simulink model "Dynamics3"  (R2023b)
settings: Solver=VariableStepAuto  StartTime=0.0  StopTime=300  RelTol=1e-3
undefined symbols (not defined in the file): env, F, iniRoll, initPitch, iniYaw, Light, MIL, tiltIni, uavParam, vIni, xGround, yGround, zGround
libraries: mbdriLib x4, slpidlib x4, aerolibasang x2, aerolibwind2 x2, shared6dof x1, sharedtransform x1, simulink x1, uavutilslib x1
(part 1 of 2)
settings Model: Creator=USER  LastModifiedBy=USER

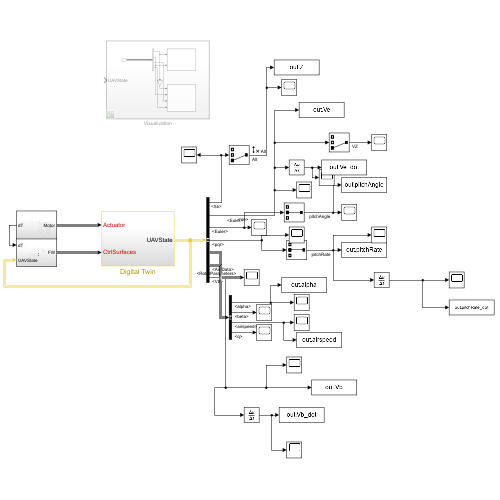
[thumbnail: Simulink's stored preview of the top-level diagram]
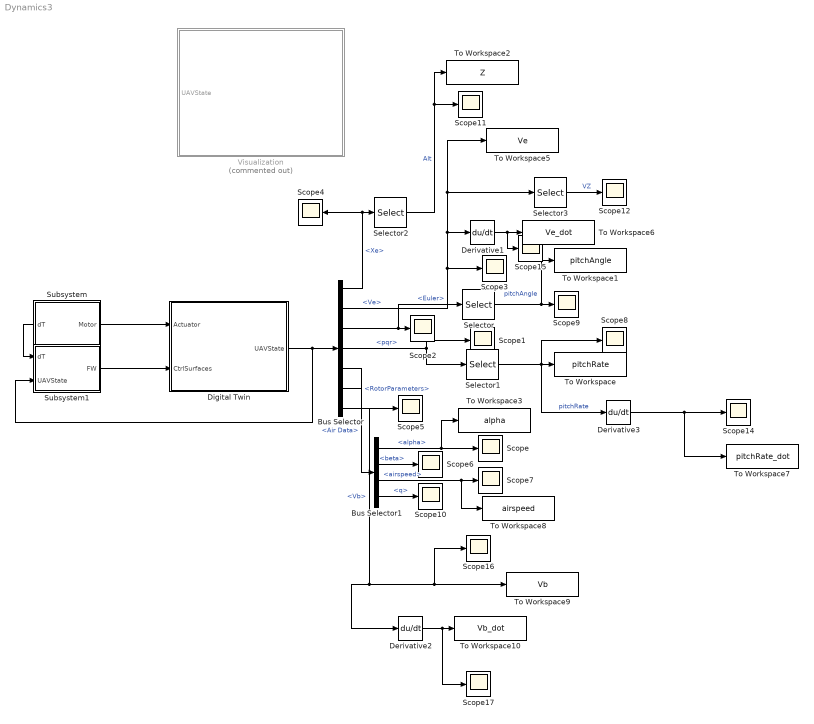
== system Dynamics3 ==
  Bus Selector : BusSelector  OutputSignals=Xe,Ve,Euler,pqr,RotorParameters,Air Data,Vb
  Bus Selector1 : BusSelector  OutputSignals=alpha,beta,airspeed,q
  Derivative1 : Derivative
  Derivative2 : Derivative
  Derivative3 : Derivative
  Digital Twin : Subsystem
  Scope{,1..12,14..17} (17 alike) : Scope
  Selector : Selector  InputPortWidth=3  IndexOptions=Index vector (dialog)  Indices=[2]  OutputSizes=1
  Selector1 : Selector  InputPortWidth=3  IndexOptions=Index vector (dialog)  Indices=[2]  OutputSizes=1
  Selector2 : Selector  InputPortWidth=3  IndexOptions=Index vector (dialog)  Indices=[3]  OutputSizes=1
  Selector3 : Selector  InputPortWidth=3  IndexOptions=Index vector (dialog)  Indices=[3]  OutputSizes=1
  Subsystem : Subsystem
      settings: PortSchema="{\"entries\":[{\"content\":{\"sides\":[{\"content\":{\"connectorIds\":[\"Out2\"]},\"type\":\"ConnectorPlacement.EquallySpacedRectSide\",\"uuid\":\"beef7808-c029-4f06-8f14-a565426224e7\"},{\"content\":{\"connectorIds\":[\"Out1\"],\"side\":\"RIGHT\"},\"type\":\"ConnectorPlacement.EquallySpacedRectSide\",\"uuid\":\"669368ed-0e99-4b02-879e-c65f4105b996\"},{\"content\":{\"side\":\"TOP\"},\"type\":\"ConnectorPlacement.EquallySpacedRectSide\",\"uuid\":\"5dd16cea-975a-4d1b-a565-9c8e907ef411\"}]},\"type\":\"ConnectorPlacement.EquallySpacedConnector\",\"uuid\":\"07c7d036-b657-434c-adc0-0d81d2cf90bb\"}],\"packageUris\":[\"http://schema.mathworks.com/mf0/Connector/R2020b\"],\"version\":\"1.0\"}"
  Subsystem1 : Subsystem
  To Workspace : ToWorkspace  VariableName=pitchRate  SampleTime=-1
  To Workspace1 : ToWorkspace  VariableName=pitchAngle  SampleTime=-1
  To Workspace10 : ToWorkspace  VariableName=Vb_dot  SampleTime=-1
  To Workspace2 : ToWorkspace  VariableName=Z  SampleTime=-1
  To Workspace3 : ToWorkspace  VariableName=alpha  SampleTime=-1
  To Workspace5 : ToWorkspace  VariableName=Ve  SampleTime=-1
  To Workspace6 : ToWorkspace  VariableName=Ve_dot  SampleTime=-1
  To Workspace7 : ToWorkspace  VariableName=pitchRate_dot  SampleTime=-1
  To Workspace8 : ToWorkspace  VariableName=airspeed  SampleTime=-1
  To Workspace9 : ToWorkspace  VariableName=Vb  SampleTime=-1
  Visualization : Subsystem  Commented=on  VariantControl=Visualization==1
  wires:
  Selector1/1 -> To Workspace/1, Scope8/1, Derivative3/1  "pitchRate"
  Bus Selector/3 -> Selector/1, Scope2/1  "<Euler>"
  Selector3/1 -> Scope12/1  "VZ"
  Bus Selector/4 -> Scope1/1, Selector1/1  "<pqr>"
  Digital Twin/1(UAVState) -> Bus Selector/1, Subsystem1/2(UAVState)
  Bus Selector1/4 -> Scope10/1  "<q>"
  Bus Selector1/3 -> To Workspace8/1, Scope7/1  "<airspeed>"
  Derivative1/1 -> Scope15/1, To Workspace6/1
  Subsystem/1(Motor) -> Digital Twin/1(Actuator)
  Bus Selector/7 -> Derivative2/1, Scope16/1, To Workspace9/1  "<Vb>"
  Bus Selector/1 -> Selector2/1, Scope4/1  "<Xe>"
  Bus Selector/5 -> Scope5/1  "<RotorParameters>"
  Bus Selector1/2 -> Scope6/1  "<beta>"
  Selector/1 -> To Workspace1/1, Scope9/1  "pitchAngle"
  Bus Selector1/1 -> To Workspace3/1, Scope/1  "<alpha>"
  Bus Selector/2 -> Derivative1/1, To Workspace5/1, Selector3/1, Scope3/1  "<Ve>"
  Selector2/1 -> To Workspace2/1, Scope11/1  "Alt"
  Derivative2/1 -> Scope17/1, To Workspace10/1
  Subsystem1/1(FW) -> Digital Twin/2(CtrlSurfaces)
  Bus Selector/6 -> Bus Selector1/1  "<Air Data>"
  Derivative3/1 -> Scope14/1, To Workspace7/1
  Subsystem/2(dT) -> Subsystem1/1(dT)

== system Dynamics3/Digital Twin ==
  Actuator : Inport
  CtrlSurfaces : Inport  Port=2
  6DOF (Euler Angles)1 : shared6dof/6DOF (Euler Angles)  units=Metric (MKS)  mtype=Fixed  rep=Euler Angles  xme_0=[xGround, yGround, zGround]  Vm_0=[vIni 0 0]  eul_0=[iniRoll initPitch iniYaw]  pm_0=[0 0 0]  mass_0=6.031  mass_e=0.5  mass_f=2.0  inertia=[uavParam.geom.Ixx 0 0; 0 uavParam.geom.Iyy 0; 0 0 uavParam.geom.Izz]  inertia_e=eye(3)  inertia_f=2*eye(3)  k_quat=1.0  vre_flag=on  abi_flag=on  aMode=0  xme_statename=''  Vm_statename=''  eul_statename=''  quat_statename=''  pm_statename=''  mass_statename=''
  Bus Selector : BusSelector  OutputSignals=RotorParameters.w1,RotorParameters.w2,RotorParameters.w3,RotorParameters.w4
  Force and Moments : Subsystem
  Ground Truth Bus : Subsystem
  Scope : Scope  NumInputPorts=4
  Terminator : Terminator
  UAVState : Outport
  wires:
  Bus Selector/4 -> Scope/4  "<w4>"
  Bus Selector/3 -> Scope/3  "<w3>"
  Bus Selector/2 -> Scope/2  "<w2>"
  Bus Selector/1 -> Scope/1  "<w1>"
  Ground Truth Bus/1(Ground Truth) -> Force and Moments/3(States), UAVState/1, Bus Selector/1  "Ground Truth"
  6DOF (Euler Angles)1/9 -> Ground Truth Bus/8(Abe)
  Force and Moments/4(AirData) -> Ground Truth Bus/10(AirData)
  Force and Moments/3(RotorParams) -> Ground Truth Bus/9(RotorParams)  "RotorParams"
  6DOF (Euler Angles)1/8 -> Ground Truth Bus/7(Abb)  "Abb"
  6DOF (Euler Angles)1/6 -> Ground Truth Bus/6(pqr)  "pqr"
  6DOF (Euler Angles)1/5 -> Ground Truth Bus/5(Vb)  "Vb"
  6DOF (Euler Angles)1/4 -> Ground Truth Bus/4(DCMbe)  "DCMbe"
  6DOF (Euler Angles)1/3 -> Ground Truth Bus/3(Euler)  "Euler"
  6DOF (Euler Angles)1/2 -> Ground Truth Bus/2(Xe)  "Xe"
  6DOF (Euler Angles)1/1 -> Ground Truth Bus/1(Ve)  "Ve"
  CtrlSurfaces/1 -> Force and Moments/2(CtrlSurfaces)
  Actuator/1 -> Force and Moments/1(Actuator)
  Force and Moments/2(M) -> 6DOF (Euler Angles)1/2
  Force and Moments/1(F) -> 6DOF (Euler Angles)1/1
  6DOF (Euler Angles)1/7 -> Terminator/1

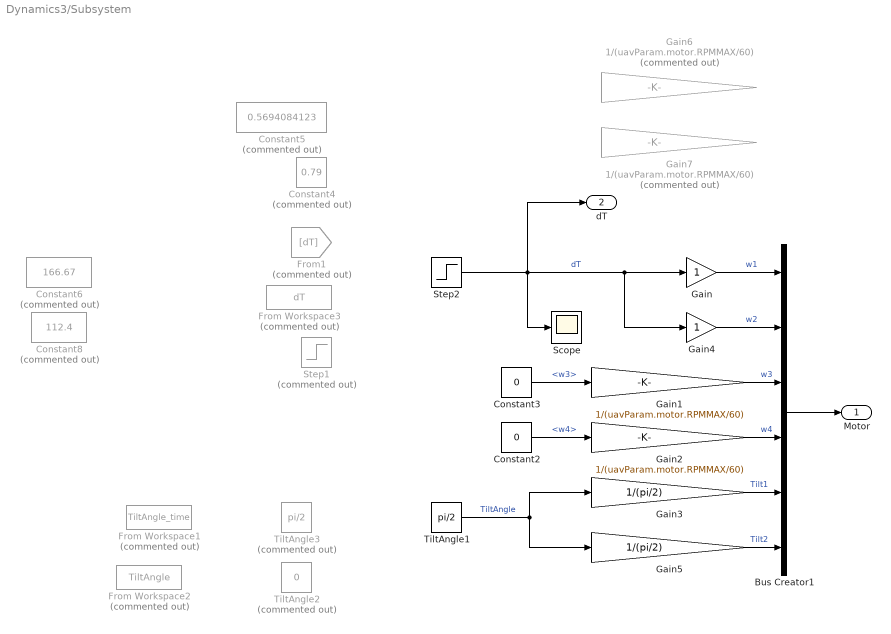
== system Dynamics3/Subsystem ==
  Bus Creator1 : BusCreator  Inputs=6  OutDataTypeStr=Bus: RotorCntrlBus
  Constant2 : Constant  Value=0
  Constant3 : Constant  Value=0
  Constant4 : Constant  Commented=on  Value=0.79
  Constant5 : Constant  Commented=on  Value=0.5694084123
  Constant6 : Constant  Commented=on  Value=166.67
  Constant8 : Constant  Commented=on  Value=112.4
  From Workspace1 : FromWorkspace  Commented=on  VariableName=TiltAngle_time
  From Workspace2 : FromWorkspace  Commented=on  VariableName=TiltAngle
  From Workspace3 : FromWorkspace  Commented=on  VariableName=dT
  From1 : From  Commented=on  GotoTag=dT
  Gain : Gain
  Gain1 : Gain  Gain=1/(uavParam.motor.RPMMAX/60)
  Gain2 : Gain  Gain=1/(uavParam.motor.RPMMAX/60)
  Gain3 : Gain  Gain=1/(pi/2)
  Gain4 : Gain
  Gain5 : Gain  Gain=1/(pi/2)
  Gain6 : Gain  Commented=on  Gain=1/(uavParam.motor.RPMMAX/60)
  Gain7 : Gain  Commented=on  Gain=1/(uavParam.motor.RPMMAX/60)
  Scope : Scope
  Step1 : Step  Commented=on  Time=100  Before=0.79  After=0.5694084123  SampleTime=0
  Step2 : Step  Time=100  Before=0.79  After=0.5694084123  SampleTime=0
  TiltAngle1 : Constant  Value=pi/2
  TiltAngle2 : Constant  Commented=on  Value=0
  TiltAngle3 : Constant  Commented=on  Value=pi/2
  Motor : Outport
  dT : Outport  Port=2
  wires:
  Constant3/1 -> Gain1/1  "<w3>"
  Constant2/1 -> Gain2/1  "<w4>"
  Gain5/1 -> Bus Creator1/6  "Tilt2"
  Gain3/1 -> Bus Creator1/5  "Tilt1"
  Gain1/1 -> Bus Creator1/3  "w3"
  Gain2/1 -> Bus Creator1/4  "w4"
  TiltAngle1/1 -> Gain5/1, Gain3/1  "TiltAngle"
  Bus Creator1/1 -> Motor/1
  Gain4/1 -> Bus Creator1/2  "w2"
  Gain/1 -> Bus Creator1/1  "w1"
  Step2/1 -> dT/1, Scope/1, Gain4/1, Gain/1  "dT"

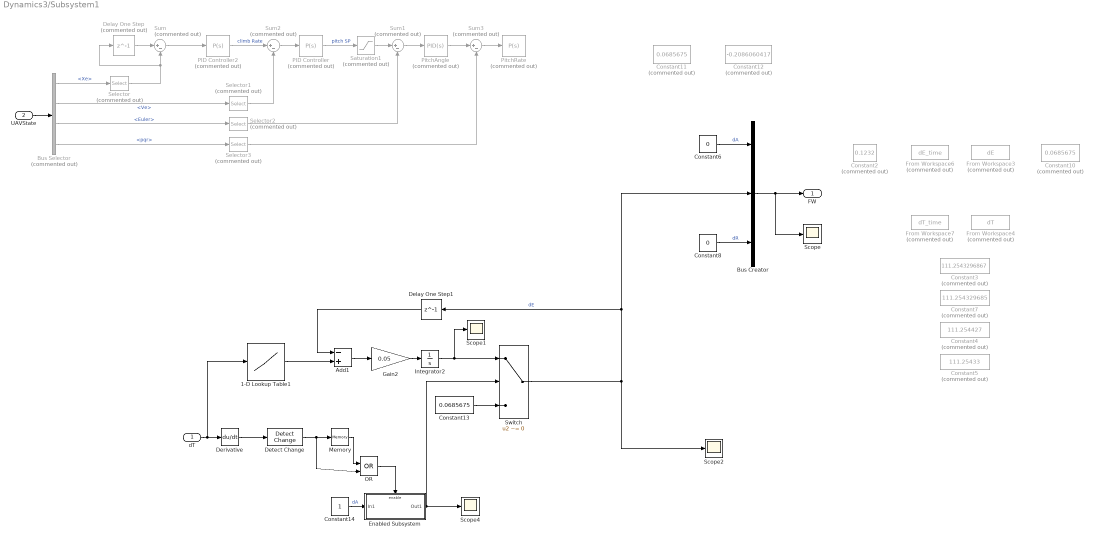
== system Dynamics3/Subsystem1 ==
  dT : Inport
  UAVState : Inport  Port=2
  1-D Lookup Table1 : Lookup_n-D  NumberOfTableDimensions=1  BreakpointsForDimension1=[0.5694084123;0.79]  Table=[-0.2086060417;0.0685675]  InternalRulePriority=Speed  RndMeth=Simplest
  Add1 : Sum  Inputs=-+
  Bus Creator : BusCreator  Inputs=3
  Bus Selector : BusSelector  Commented=on  OutputSignals=Xe,Ve,Euler,pqr
  Constant10 : Constant  Commented=on  Value=0.0685675
  Constant11 : Constant  Commented=on  Value=0.0685675
  Constant12 : Constant  Commented=on  Value=-0.2086060417
  Constant13 : Constant  Value=0.0685675
  Constant14 : Constant
  Constant2 : Constant  Commented=on  Value=0.1232
  Constant3 : Constant  Commented=on  Value=111.2543296867
  Constant4 : Constant  Commented=on  Value=111.254427
  Constant5 : Constant  Commented=on  Value=111.25433
  Constant6 : Constant  Value=0
  Constant7 : Constant  Commented=on  Value=111.254329685
  Constant8 : Constant  Value=0
  Delay One Step : Delay  Commented=on  DelayLength=1
  Delay One Step1 : Delay  DelayLength=1
  Derivative : Derivative
  Detect Change : simulink/Logic and Bit Operations/Detect Change  vinit=0  OutDataTypeStr=boolean
  Enabled Subsystem : Subsystem  TreatAsAtomicUnit=on
  From Workspace3 : FromWorkspace  Commented=on  VariableName=dE  OutDataTypeStr=double
  From Workspace4 : FromWorkspace  Commented=on  VariableName=dT  OutDataTypeStr=double
  From Workspace6 : FromWorkspace  Commented=on  VariableName=dE_time
  From Workspace7 : FromWorkspace  Commented=on  VariableName=dT_time
  Gain2 : Gain  Gain=0.05
  Integrator2 : Integrator
  Memory : Memory
  OR : Logic  Operator=OR  IconShape=distinctive  AllPortsSameDT=off  OutDataTypeStr=boolean
  PID Controller : slpidlib/PID Controller  Commented=on  Controller=P  Form=Parallel  TimeDomain=Continuous-time  UseExternalTs=off  SampleTime=-1  IntegratorMethod=Forward Euler  FilterMethod=Forward Euler  ControllerParametersSource=internal  P=0.253636873440471  I=1  UseKiTs=off  D=0  N=100  UseFilter=on  TunerSelectOption=Transfer Function Based (PID Tuner App)  InitialConditionSource=internal  InitialConditionForIntegrator=0  InitialConditionForFilter=0  DifferentiatorICPrevScaledInput=0  ExternalReset=none  TrackingMode=off  Kt=1  LimitOutput=off  SatLimitsSource=internal  UpperSaturationLimit=inf  LowerSaturationLimit=-inf  LinearizeAsGain=on  AntiWindupMode=none  Kb=1  LimitIntegrator=off  UpperIntegratorSaturationLimit=inf  LowerIntegratorSaturationLimit=-inf  POutMin=[]  POutMax=[]  IOutMin=[]  IOutMax=[]  DOutMin=[]  DOutMax=[]  NOutMin=[]  NOutMax=[]  SumOutMin=[]  SumOutMax=[]  SaturationOutMin=[]  SaturationOutMax=[]  PParamMin=[]  PParamMax=[]  IParamMin=[]  IParamMax=[]  DParamMin=[]  DParamMax=[]  NParamMin=[]  NParamMax=[]  KbParamMin=[]  KbParamMax=[]  KtParamMin=[]  KtParamMax=[]  KbOutMin=[]  KbOutMax=[]  KtOutMin=[]  KtOutMax=[]  IntegratorOutMin=[]  IntegratorOutMax=[]  FilterOutMin=[]  FilterOutMax=[]  SumI1OutMin=[]  SumI1OutMax=[]  SumI2OutMin=[]  SumI2OutMax=[]  SumI3OutMin=[]  SumI3OutMax=[]  SumI4OutMin=[]  SumI4OutMax=[]  SumDOutMin=[]  SumDOutMax=[]  DifferentiatorOutMin=[]  DifferentiatorOutMax=[]  FilterDiffOutCoefMin=[]  FilterDiffOutCoefMax=[]  ReciprocalOutMin=[]  ReciprocalOutMax=[]  SumDenOutMin=[]  SumDenOutMax=[]  SumNumOutMin=[]  SumNumOutMax=[]  DivideOutMin=[]  DivideOutMax=[]  UdiffTsProdOutMin=[]  UdiffTsProdOutMax=[]  NTsProdOutMin=[]  NTsProdOutMax=[]  UintegralTsProdOutMin=[]  UintegralTsProdOutMax=[]  UngainTsProdOutMin=[]  UngainTsProdOutMax=[]  ClampingZeroOutDataTypeStr=Inherit: Inherit via back propagation  ClampingZeroOutMin=[]  ClampingZeroOutMax=[]  FilterDenConstantOutDataTypeStr=Inherit: Inherit via back propagation  FilterDenConstantOutMin=[]  FilterDenConstantOutMax=[]  PCopyOutDataTypeStr=Inherit: Inherit via back propagation  PCopyOutMin=[]  PCopyOutMax=[]  NCopyOutDataTypeStr=Inherit: Inherit via back propagation  NCopyOutMin=[]  NCopyOutMax=[]  IntegratorContinuousStateAttributes=''  IntegratorStateMustResolveToSignalObject=off  IntegratorRTWStateStorageClass=Auto  FilterContinuousStateAttributes=''  FilterStateMustResolveToSignalObject=off  FilterRTWStateStorageClass=Auto  ParallelPVariant=InternalParameters  IdealPVariant=Disabled  IVariant=Disabled  DVariant=Disabled  IntegratorVariant=Disabled  SatVariant=Disabled  AWVariant=Disabled  PCopyVariant=Disabled  TRVariant=Disabled  FdbkBlocksVariant=Forward  IdealPFdbkVariant=Disabled  SatFdbkVariant=Disabled  DerivativeFilterVariant=Disabled  NVariant=Disabled  NCopyVariant=Disabled_SignalSpec  FilterICVariant=Disabled  IntegratorICVariant=Disabled  ExternalResetVariant=Disabled  TRSumVariant=Passthrough  SumFdbkVariant=Disabled  SumVariant=Passthrough_P  TsampFilterVariant=InternalTs  TsampNgainVariant=Passthrough  TsampIntegralVariant=Disabled_SignalSpec  ExternalSaturationOutDataTypeStr=Inherit: Same as second input
  PID Controller2 : slpidlib/PID Controller  Commented=on  Controller=P  Form=Parallel  TimeDomain=Continuous-time  UseExternalTs=off  SampleTime=-1  IntegratorMethod=Forward Euler  FilterMethod=Forward Euler  ControllerParametersSource=internal  P=100  I=1  UseKiTs=off  D=0  N=100  UseFilter=on  TunerSelectOption=Transfer Function Based (PID Tuner App)  InitialConditionSource=internal  InitialConditionForIntegrator=0  InitialConditionForFilter=0  DifferentiatorICPrevScaledInput=0  ExternalReset=none  TrackingMode=off  Kt=1  LimitOutput=off  SatLimitsSource=internal  UpperSaturationLimit=inf  LowerSaturationLimit=-inf  LinearizeAsGain=on  AntiWindupMode=none  Kb=1  LimitIntegrator=off  UpperIntegratorSaturationLimit=inf  LowerIntegratorSaturationLimit=-inf  POutMin=[]  POutMax=[]  IOutMin=[]  IOutMax=[]  DOutMin=[]  DOutMax=[]  NOutMin=[]  NOutMax=[]  SumOutMin=[]  SumOutMax=[]  SaturationOutMin=[]  SaturationOutMax=[]  PParamMin=[]  PParamMax=[]  IParamMin=[]  IParamMax=[]  DParamMin=[]  DParamMax=[]  NParamMin=[]  NParamMax=[]  KbParamMin=[]  KbParamMax=[]  KtParamMin=[]  KtParamMax=[]  KbOutMin=[]  KbOutMax=[]  KtOutMin=[]  KtOutMax=[]  IntegratorOutMin=[]  IntegratorOutMax=[]  FilterOutMin=[]  FilterOutMax=[]  SumI1OutMin=[]  SumI1OutMax=[]  SumI2OutMin=[]  SumI2OutMax=[]  SumI3OutMin=[]  SumI3OutMax=[]  SumI4OutMin=[]  SumI4OutMax=[]  SumDOutMin=[]  SumDOutMax=[]  DifferentiatorOutMin=[]  DifferentiatorOutMax=[]  FilterDiffOutCoefMin=[]  FilterDiffOutCoefMax=[]  ReciprocalOutMin=[]  ReciprocalOutMax=[]  SumDenOutMin=[]  SumDenOutMax=[]  SumNumOutMin=[]  SumNumOutMax=[]  DivideOutMin=[]  DivideOutMax=[]  UdiffTsProdOutMin=[]  UdiffTsProdOutMax=[]  NTsProdOutMin=[]  NTsProdOutMax=[]  UintegralTsProdOutMin=[]  UintegralTsProdOutMax=[]  UngainTsProdOutMin=[]  UngainTsProdOutMax=[]  ClampingZeroOutDataTypeStr=Inherit: Inherit via back propagation  ClampingZeroOutMin=[]  ClampingZeroOutMax=[]  FilterDenConstantOutDataTypeStr=Inherit: Inherit via back propagation  FilterDenConstantOutMin=[]  FilterDenConstantOutMax=[]  PCopyOutDataTypeStr=Inherit: Inherit via back propagation  PCopyOutMin=[]  PCopyOutMax=[]  NCopyOutDataTypeStr=Inherit: Inherit via back propagation  NCopyOutMin=[]  NCopyOutMax=[]  IntegratorContinuousStateAttributes=''  IntegratorStateMustResolveToSignalObject=off  IntegratorRTWStateStorageClass=Auto  FilterContinuousStateAttributes=''  FilterStateMustResolveToSignalObject=off  FilterRTWStateStorageClass=Auto  ParallelPVariant=InternalParameters  IdealPVariant=Disabled  IVariant=Disabled  DVariant=Disabled  IntegratorVariant=Disabled  SatVariant=Disabled  AWVariant=Disabled  PCopyVariant=Disabled  TRVariant=Disabled  FdbkBlocksVariant=Forward  IdealPFdbkVariant=Disabled  SatFdbkVariant=Disabled  DerivativeFilterVariant=Disabled  NVariant=Disabled  NCopyVariant=Disabled_SignalSpec  FilterICVariant=Disabled  IntegratorICVariant=Disabled  ExternalResetVariant=Disabled  TRSumVariant=Passthrough  SumFdbkVariant=Disabled  SumVariant=Passthrough_P  TsampFilterVariant=InternalTs  TsampNgainVariant=Passthrough  TsampIntegralVariant=Disabled_SignalSpec  ExternalSaturationOutDataTypeStr=Inherit: Same as second input
  PitchAngle : slpidlib/PID Controller  Commented=on  Controller=PID  Form=Parallel  TimeDomain=Continuous-time  UseExternalTs=off  SampleTime=-1  IntegratorMethod=Forward Euler  FilterMethod=Forward Euler  ControllerParametersSource=internal  P=17.6399272009125  I=10.1914925604101  UseKiTs=off  D=1.4272793655692  N=0.16530941788163  UseFilter=on  TunerSelectOption=Transfer Function Based (PID Tuner App)  InitialConditionSource=internal  InitialConditionForIntegrator=0  InitialConditionForFilter=0  DifferentiatorICPrevScaledInput=0  ExternalReset=none  TrackingMode=off  Kt=1  LimitOutput=off  SatLimitsSource=internal  UpperSaturationLimit=inf  LowerSaturationLimit=-inf  LinearizeAsGain=on  AntiWindupMode=none  Kb=1  LimitIntegrator=off  UpperIntegratorSaturationLimit=inf  LowerIntegratorSaturationLimit=-inf  POutMin=[]  POutMax=[]  IOutMin=[]  IOutMax=[]  DOutMin=[]  DOutMax=[]  NOutMin=[]  NOutMax=[]  SumOutMin=[]  SumOutMax=[]  SaturationOutMin=[]  SaturationOutMax=[]  PParamMin=[]  PParamMax=[]  IParamMin=[]  IParamMax=[]  DParamMin=[]  DParamMax=[]  NParamMin=[]  NParamMax=[]  KbParamMin=[]  KbParamMax=[]  KtParamMin=[]  KtParamMax=[]  KbOutMin=[]  KbOutMax=[]  KtOutMin=[]  KtOutMax=[]  IntegratorOutMin=[]  IntegratorOutMax=[]  FilterOutMin=[]  FilterOutMax=[]  SumI1OutMin=[]  SumI1OutMax=[]  SumI2OutMin=[]  SumI2OutMax=[]  SumI3OutMin=[]  SumI3OutMax=[]  SumI4OutMin=[]  SumI4OutMax=[]  SumDOutMin=[]  SumDOutMax=[]  DifferentiatorOutMin=[]  DifferentiatorOutMax=[]  FilterDiffOutCoefMin=[]  FilterDiffOutCoefMax=[]  ReciprocalOutMin=[]  ReciprocalOutMax=[]  SumDenOutMin=[]  SumDenOutMax=[]  SumNumOutMin=[]  SumNumOutMax=[]  DivideOutMin=[]  DivideOutMax=[]  UdiffTsProdOutMin=[]  UdiffTsProdOutMax=[]  NTsProdOutMin=[]  NTsProdOutMax=[]  UintegralTsProdOutMin=[]  UintegralTsProdOutMax=[]  UngainTsProdOutMin=[]  UngainTsProdOutMax=[]  ClampingZeroOutDataTypeStr=Inherit: Inherit via back propagation  ClampingZeroOutMin=[]  ClampingZeroOutMax=[]  FilterDenConstantOutDataTypeStr=Inherit: Inherit via back propagation  FilterDenConstantOutMin=[]  FilterDenConstantOutMax=[]  PCopyOutDataTypeStr=Inherit: Inherit via back propagation  PCopyOutMin=[]  PCopyOutMax=[]  NCopyOutDataTypeStr=Inherit: Inherit via back propagation  NCopyOutMin=[]  NCopyOutMax=[]  IntegratorContinuousStateAttributes=''  IntegratorStateMustResolveToSignalObject=off  IntegratorRTWStateStorageClass=Auto  FilterContinuousStateAttributes=''  FilterStateMustResolveToSignalObject=off  FilterRTWStateStorageClass=Auto  ParallelPVariant=InternalParameters  IdealPVariant=Disabled  IVariant=InternalParameters  DVariant=InternalParameters  IntegratorVariant=Continuous  SatVariant=Disabled  AWVariant=Passthrough  PCopyVariant=Disabled  TRVariant=Disabled  FdbkBlocksVariant=Forward  IdealPFdbkVariant=Disabled  SatFdbkVariant=Disabled  DerivativeFilterVariant=ContFilter  NVariant=InternalParameters  NCopyVariant=Disabled  FilterICVariant=InternalICsFilter  IntegratorICVariant=InternalICs  ExternalResetVariant=Disabled  TRSumVariant=Passthrough  SumFdbkVariant=Disabled  SumVariant=Sum_PID  TsampFilterVariant=InternalTs  TsampNgainVariant=Passthrough  TsampIntegralVariant=Disabled_SignalSpec  ExternalSaturationOutDataTypeStr=Inherit: Same as second input
  PitchRate : slpidlib/PID Controller  Commented=on  Controller=P  Form=Parallel  TimeDomain=Continuous-time  UseExternalTs=off  SampleTime=-1  IntegratorMethod=Forward Euler  FilterMethod=Forward Euler  ControllerParametersSource=internal  P=0.198532533167891  I=1  UseKiTs=off  D=0  N=100  UseFilter=on  TunerSelectOption=Transfer Function Based (PID Tuner App)  InitialConditionSource=internal  InitialConditionForIntegrator=0  InitialConditionForFilter=0  DifferentiatorICPrevScaledInput=0  ExternalReset=none  TrackingMode=off  Kt=1  LimitOutput=off  SatLimitsSource=internal  UpperSaturationLimit=inf  LowerSaturationLimit=-inf  LinearizeAsGain=on  AntiWindupMode=none  Kb=1  LimitIntegrator=off  UpperIntegratorSaturationLimit=inf  LowerIntegratorSaturationLimit=-inf  POutMin=[]  POutMax=[]  IOutMin=[]  IOutMax=[]  DOutMin=[]  DOutMax=[]  NOutMin=[]  NOutMax=[]  SumOutMin=[]  SumOutMax=[]  SaturationOutMin=[]  SaturationOutMax=[]  PParamMin=[]  PParamMax=[]  IParamMin=[]  IParamMax=[]  DParamMin=[]  DParamMax=[]  NParamMin=[]  NParamMax=[]  KbParamMin=[]  KbParamMax=[]  KtParamMin=[]  KtParamMax=[]  KbOutMin=[]  KbOutMax=[]  KtOutMin=[]  KtOutMax=[]  IntegratorOutMin=[]  IntegratorOutMax=[]  FilterOutMin=[]  FilterOutMax=[]  SumI1OutMin=[]  SumI1OutMax=[]  SumI2OutMin=[]  SumI2OutMax=[]  SumI3OutMin=[]  SumI3OutMax=[]  SumI4OutMin=[]  SumI4OutMax=[]  SumDOutMin=[]  SumDOutMax=[]  DifferentiatorOutMin=[]  DifferentiatorOutMax=[]  FilterDiffOutCoefMin=[]  FilterDiffOutCoefMax=[]  ReciprocalOutMin=[]  ReciprocalOutMax=[]  SumDenOutMin=[]  SumDenOutMax=[]  SumNumOutMin=[]  SumNumOutMax=[]  DivideOutMin=[]  DivideOutMax=[]  UdiffTsProdOutMin=[]  UdiffTsProdOutMax=[]  NTsProdOutMin=[]  NTsProdOutMax=[]  UintegralTsProdOutMin=[]  UintegralTsProdOutMax=[]  UngainTsProdOutMin=[]  UngainTsProdOutMax=[]  ClampingZeroOutDataTypeStr=Inherit: Inherit via back propagation  ClampingZeroOutMin=[]  ClampingZeroOutMax=[]  FilterDenConstantOutDataTypeStr=Inherit: Inherit via back propagation  FilterDenConstantOutMin=[]  FilterDenConstantOutMax=[]  PCopyOutDataTypeStr=Inherit: Inherit via back propagation  PCopyOutMin=[]  PCopyOutMax=[]  NCopyOutDataTypeStr=Inherit: Inherit via back propagation  NCopyOutMin=[]  NCopyOutMax=[]  IntegratorContinuousStateAttributes=''  IntegratorStateMustResolveToSignalObject=off  IntegratorRTWStateStorageClass=Auto  FilterContinuousStateAttributes=''  FilterStateMustResolveToSignalObject=off  FilterRTWStateStorageClass=Auto  ParallelPVariant=InternalParameters  IdealPVariant=Disabled  IVariant=Disabled  DVariant=Disabled  IntegratorVariant=Disabled  SatVariant=Disabled  AWVariant=Disabled  PCopyVariant=Disabled  TRVariant=Disabled  FdbkBlocksVariant=Forward  IdealPFdbkVariant=Disabled  SatFdbkVariant=Disabled  DerivativeFilterVariant=Disabled  NVariant=Disabled  NCopyVariant=Disabled_SignalSpec  FilterICVariant=Disabled  IntegratorICVariant=Disabled  ExternalResetVariant=Disabled  TRSumVariant=Passthrough  SumFdbkVariant=Disabled  SumVariant=Passthrough_P  TsampFilterVariant=InternalTs  TsampNgainVariant=Passthrough  TsampIntegralVariant=Disabled_SignalSpec  ExternalSaturationOutDataTypeStr=Inherit: Same as second input
  Saturation1 : Saturate  Commented=on  UpperLimit=0.17  LowerLimit=-0.17
  Scope{,1..2,4} (4 alike) : Scope
  Selector : Selector  Commented=on  InputPortWidth=3  IndexOptions=Index vector (dialog)  Indices=3  OutputSizes=1
  Selector1 : Selector  Commented=on  InputPortWidth=3  IndexOptions=Index vector (dialog)  Indices=3  OutputSizes=1
  Selector2 : Selector  Commented=on  InputPortWidth=3  IndexOptions=Index vector (dialog)  Indices=2  OutputSizes=1
  Selector3 : Selector  Commented=on  InputPortWidth=3  IndexOptions=Index vector (dialog)  Indices=2  OutputSizes=1
  Sum{,1..3} (4 alike) : Sum  Commented=on  Inputs=|+-
  Switch : Switch  Criteria=u2 ~= 0  SaturateOnIntegerOverflow=off  InputSameDT=off
  FW : Outport
  wires:
  Constant6/1 -> Bus Creator/1  "dA"
  Constant8/1 -> Bus Creator/3  "dR"
  Bus Creator/1 -> Scope/1, FW/1
  Delay One Step/1 -> Sum/1
  Selector/1 -> Delay One Step/1, Sum/2
  Sum/1 -> PID Controller2/1
  Bus Selector/1 -> Selector/1  "<Xe>"
  PID Controller/1 -> Saturation1/1  "pitch SP"
  Bus Selector/2 -> Selector1/1  "<Ve>"
  Selector1/1 -> Sum2/2
  PID Controller2/1 -> Sum2/1  "climb Rate"
  Sum2/1 -> PID Controller/1
  Bus Selector/3 -> Selector2/1  "<Euler>"
  Bus Selector/4 -> Selector3/1  "<pqr>"
  Saturation1/1 -> Sum1/1
  Sum1/1 -> PitchAngle/1
  PitchAngle/1 -> Sum3/1
  Sum3/1 -> PitchRate/1
  Selector2/1 -> Sum1/2
  Selector3/1 -> Sum3/2
  Switch/1 -> Delay One Step1/1, Bus Creator/2, Scope2/1  "dE"
  Enabled Subsystem/1(Out1) -> Switch/2, Scope4/1
  Derivative/1 -> Detect Change/1
  Detect Change/1 -> Memory/1, OR/2
  Memory/1 -> OR/1
  OR/1 -> Enabled Subsystem/Enable
  Constant13/1 -> Switch/3
  Constant14/1 -> Enabled Subsystem/1(In1)  "dA"
  UAVState/1 -> Bus Selector/1
  Gain2/1 -> Integrator2/1
  Integrator2/1 -> Scope1/1, Switch/1
  Add1/1 -> Gain2/1
  1-D Lookup Table1/1 -> Add1/2
  dT/1 -> 1-D Lookup Table1/1, Derivative/1
  Delay One Step1/1 -> Add1/1

== system Dynamics3/Visualization ==
  UAVState : Inport
  Bus Selector : BusSelector  OutputSignals=Xe,q,RotorParameters.Rotor A,RotorParameters.Rotor B
  Gain : Gain  Gain=0
  Subsystem : Subsystem
  Trajectory : uavutilslib/UAV Animation  UAVType=FixedWing  UAVSize=5  InertialZDirection=Down  SampleTime=0.1
  wires:
  Bus Selector/4 -> Subsystem/4(RotorB)  "<Rotor B>"
  Bus Selector/3 -> Subsystem/3(RotorA)  "<Rotor A>"
  UAVState/1 -> Bus Selector/1
  Gain/1 -> Subsystem/1(<Xe>)
  Bus Selector/1 -> Gain/1, Trajectory/1  "<Xe>"
  Bus Selector/2 -> Trajectory/2, Subsystem/2(<q>)  "<q>"

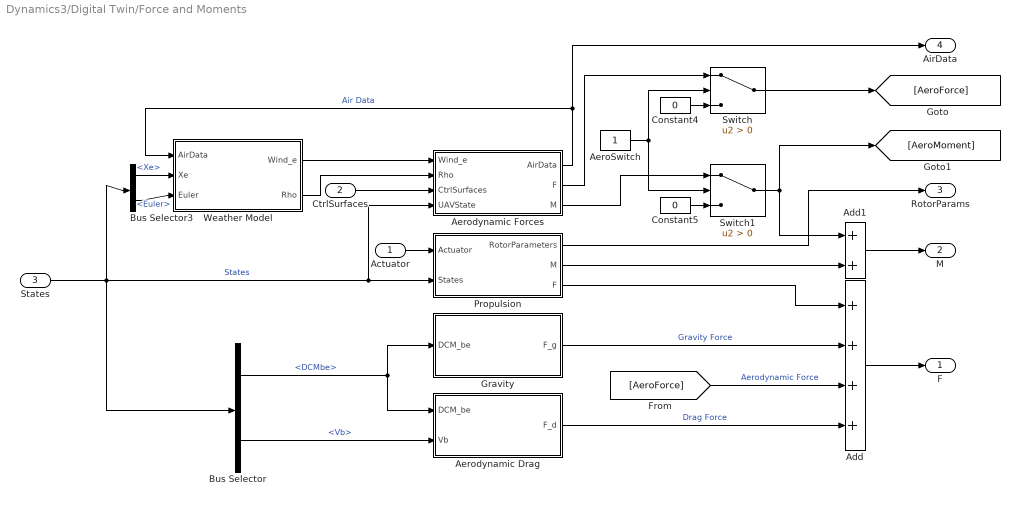
== system Dynamics3/Digital Twin/Force and Moments ==
  Actuator : Inport
  CtrlSurfaces : Inport  Port=2
  States : Inport  Port=3
  Add : Sum  Inputs=++++
  Add1 : Sum
  AeroSwitch : Constant
  Aerodynamic Drag : Subsystem
  Aerodynamic Forces : Subsystem
  Bus Selector : BusSelector  OutputSignals=DCMbe,Vb
  Bus Selector3 : BusSelector  OutputSignals=Xe,Euler
  Constant4 : Constant  Value=0
  Constant5 : Constant  Value=0
  Gravity : Subsystem
  Propulsion : Subsystem
  Switch : Switch  Criteria=u2 > Threshold  SaturateOnIntegerOverflow=off  InputSameDT=off
  Switch1 : Switch  Criteria=u2 > Threshold  SaturateOnIntegerOverflow=off  InputSameDT=off
  Weather Model : Subsystem  Variant=on  VariantControl=Weather Model
  F : Outport
  M : Outport  Port=2
  RotorParams : Outport  Port=3
  AirData : Outport  Port=4
  wires:
  Weather Model/2(Rho) -> Aerodynamic Forces/2(Rho)
  Weather Model/1(Wind_e) -> Aerodynamic Forces/1(Wind_e)
  Bus Selector3/2 -> Weather Model/3(Euler)  "<Euler>"
  Bus Selector3/1 -> Weather Model/2(Xe)  "<Xe>"
  Aerodynamic Forces/1(AirData) -> Weather Model/1(AirData), AirData/1  "Air Data"
  Propulsion/1(RotorParameters) -> RotorParams/1
  Actuator/1 -> Propulsion/1(Actuator)
  Aerodynamic Forces/3(M) -> Switch1/1
  Switch1/1 -> [AeroMoment], Add1/1
  Constant5/1 -> Switch1/3
  AeroSwitch/1 -> Switch1/2, Switch/2
  Constant4/1 -> Switch/3
  Switch/1 -> [AeroForce]
  Aerodynamic Forces/2(F) -> Switch/1
  [AeroForce] -> Add/3  "Aerodynamic Force"
  Propulsion/2(M) -> Add1/2
  Add1/1 -> M/1
  CtrlSurfaces/1 -> Aerodynamic Forces/3(CtrlSurfaces)
  States/1 -> Propulsion/2(States), Aerodynamic Forces/4(UAVState), Bus Selector/1, Bus Selector3/1  "States"
  Add/1 -> F/1
  Bus Selector/2 -> Aerodynamic Drag/2(Vb)  "<Vb>"
  Aerodynamic Drag/1(F_d) -> Add/4  "Drag Force"
  Gravity/1(F_g) -> Add/2  "Gravity Force"
  Propulsion/3(F) -> Add/1
  Bus Selector/1 -> Aerodynamic Drag/1(DCM_be), Gravity/1(DCM_be)  "<DCMbe>"

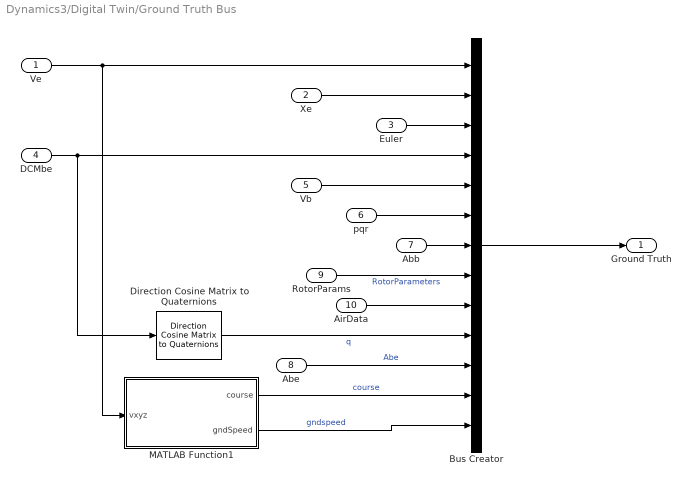
== system Dynamics3/Digital Twin/Ground Truth Bus ==
  Ve : Inport
  Xe : Inport  Port=2
  Euler : Inport  Port=3
  DCMbe : Inport  Port=4
  Vb : Inport  Port=5
  pqr : Inport  Port=6
  Abb : Inport  Port=7
  Abe : Inport  Port=8
  RotorParams : Inport  Port=9
  AirData : Inport  Port=10
  Bus Creator : BusCreator  Inputs=13
  Direction Cosine Matrix to Quaternions : sharedtransform/Direction Cosine Matrix  to Quaternions  aMode=0  action=None  tolerance=eps(2)
      settings: LibrarySourceBlock=|
      | aerolibtransform2/Direction Cosine Matrix
      | to Quaternions
  MATLAB Function1 : MATLAB Function  TreatAsAtomicUnit=on
  Ground Truth : Outport
  wires:
  Ve/1 -> Bus Creator/1, MATLAB Function1/1(vxyz)
  MATLAB Function1/1(course) -> Bus Creator/12  "course"
  MATLAB Function1/2(gndSpeed) -> Bus Creator/13  "gndspeed"
  Abe/1 -> Bus Creator/11  "Abe"
  RotorParams/1 -> Bus Creator/8  "RotorParameters"
  Direction Cosine Matrix to Quaternions/1 -> Bus Creator/10  "q"
  AirData/1 -> Bus Creator/9
  Abb/1 -> Bus Creator/7
  Vb/1 -> Bus Creator/5
  Euler/1 -> Bus Creator/3
  DCMbe/1 -> Bus Creator/4, Direction Cosine Matrix to Quaternions/1
  Bus Creator/1 -> Ground Truth/1
  Xe/1 -> Bus Creator/2
  pqr/1 -> Bus Creator/6

== system Dynamics3/Subsystem1/Enabled Subsystem ==
  In1 : Inport
  Enable : EnablePort
  Out1 : Outport
  wires:
  In1/1 -> Out1/1

== system Dynamics3/Visualization/Subsystem ==
  <Xe> : Inport
  <q> : Inport  Port=2
  RotorA : Inport  Port=3
  RotorB : Inport  Port=4
  Constant : Constant  Commented=on  Value=0
  Constant1 : Constant  Commented=on  Value=0
  Gain : Gain  Gain=0
  Gain1 : Gain  Gain=-1
  Gain2 : Gain  Gain=-1
  MATLAB System : MATLABSystem  System=exampleHelperTiltRotorAnimator  SampleTime=0.05
      mask Type: exampleHelperTiltRotorAnimator
      mask Display:
      | disp('exampleHelperTiltRotorAnimator');
      | port_label('input',1,'position');
      | port_label('input',2,'orientation');
      | port_label('input',3,'rotorAngles');
  Mux : Mux  Inputs=2
  Reshape : Reshape  OutputDimensionality=Customize  OutputDimensions=[1,4]
  Reshape1 : Reshape  OutputDimensionality=Customize  OutputDimensions=[1,2]
  Reshape2 : Reshape  OutputDimensionality=Customize  OutputDimensions=[1,3]
  wires:
  Gain/1 -> Reshape2/1
  Reshape/1 -> MATLAB System/2
  Reshape2/1 -> MATLAB System/1
  <q>/1 -> Reshape/1
  RotorB/1 -> Gain2/1
  Constant/1 -> ?
  <Xe>/1 -> Gain/1
  RotorA/1 -> Gain1/1
  Mux/1 -> Reshape1/1
  Reshape1/1 -> MATLAB System/3
  Gain2/1 -> Mux/2
  Constant1/1 -> ?
  Gain1/1 -> Mux/1

== system Dynamics3/Digital Twin/Force and Moments/Aerodynamic Drag ==
  DCM_be : Inport
  Vb : Inport  Port=2
  Constant : Constant  Value=[0,0,0]
  Constant1 : Constant  Value=uavParam.aero.dragCoeffMov
  calcDragVector : MATLAB Function  TreatAsAtomicUnit=on
  gain : Gain  Gain=-1
  relative air velocity (body frame) : Sum
  wind (body frame) : Product  Multiplication=Matrix(*)
  F_d : Outport
  wires:
  wind (body frame)/1 -> relative air velocity (body frame)/1
  Constant/1 -> wind (body frame)/2
  DCM_be/1 -> wind (body frame)/1
  Constant1/1 -> calcDragVector/2(dragCoeff)
  gain/1 -> relative air velocity (body frame)/2
  relative air velocity (body frame)/1 -> calcDragVector/1(airVel)
  calcDragVector/1(dragVec) -> F_d/1
  Vb/1 -> gain/1

== system Dynamics3/Digital Twin/Force and Moments/Aerodynamic Forces ==
  Wind_e : Inport
  Rho : Inport  Port=2
  CtrlSurfaces : Inport  Port=3
  UAVState : Inport  Port=4
  Bus Selector2 : BusSelector  OutputSignals=Ve,Euler,pqr
  Compute Air Data : Subsystem  TreatAsAtomicUnit=on  VariantControl=use_aerospace_blocks == 1
  Compute Body Frame Forces and Moments : Subsystem
  Rotate Vw : Subsystem
  Vair : Sum  Inputs=-+  InputSameDT=on  SaturateOnIntegerOverflow=on  OutDataTypeStr=Inherit: Same as first input
  AirData : Outport  VectorParamsAs1DForOutWhenUnconnected=off
  F : Outport  Port=2
  M : Outport  Port=3
  wires:
  Vair/1 -> Rotate Vw/1(Vw)
  Bus Selector2/2 -> Rotate Vw/2(Euler)  "<Euler>"
  Rho/1 -> Compute Air Data/2(Rho)
  Rotate Vw/1(Vb) -> Compute Air Data/1(Vb)
  Compute Body Frame Forces and Moments/2(M_b) -> M/1
  Bus Selector2/3 -> Compute Body Frame Forces and Moments/3(p,q,r)  "<pqr>"
  Compute Air Data/1(AirData) -> Compute Body Frame Forces and Moments/1(AirData), AirData/1
  CtrlSurfaces/1 -> Compute Body Frame Forces and Moments/2(CtrlSurfaces)
  Wind_e/1 -> Vair/1
  Compute Body Frame Forces and Moments/1(F_b) -> F/1
  UAVState/1 -> Bus Selector2/1
  Bus Selector2/1 -> Vair/2  "<Ve>"

== system Dynamics3/Digital Twin/Force and Moments/Gravity ==
  DCM_be : Inport
  Constant : Constant  Value=[0 0 uavParam.aero.g]'
  Gain : Gain  Gain=uavParam.geom.mass
  Matrix Multiply : Product  Multiplication=Matrix(*)
  F_g : Outport
  wires:
  Gain/1 -> F_g/1
  DCM_be/1 -> Matrix Multiply/1
  Constant/1 -> Matrix Multiply/2
  Matrix Multiply/1 -> Gain/1

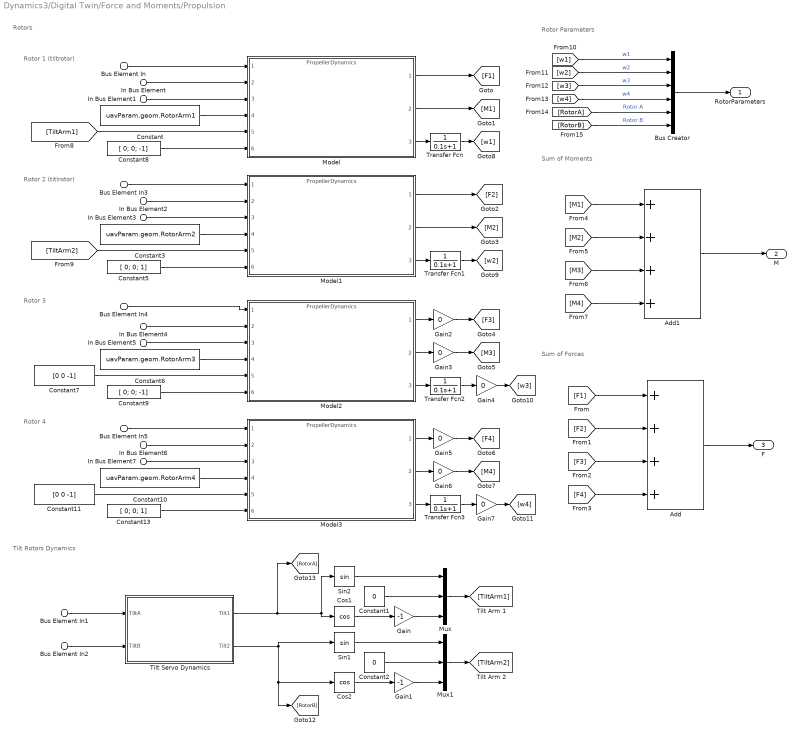
== system Dynamics3/Digital Twin/Force and Moments/Propulsion ==
  note: Rotor Parameters
  note: Sum of Forces
  note: Rotor 4
  note: Rotor 3
  note: Rotor 2
      | (titlrotor)
  note: Rotors
  note: Rotor 1
      | (tiltrotor)
  note: Sum of Moments
  note: Tilt Rotors Dynamics
  Bus Element In : Inport  PortName=Actuator  Element=w1
  Bus Element In1 : Inport  PortName=Actuator  Element=Tilt1
  Bus Element In2 : Inport  PortName=Actuator  Element=Tilt2
  Bus Element In3 : Inport  PortName=Actuator  Element=w2
  Bus Element In5 : Inport  PortName=Actuator  Element=w4
  Bus Element In4 : Inport  PortName=Actuator  Element=w3
  In Bus Element{,2,4,6} (4 alike) : Inport  Port=2  PortName=States  Element=Vb
  In Bus Element{1,3,5,7} (4 alike) : Inport  Port=2  PortName=States  Element=pqr
  Add : Sum  Inputs=++++
  Add1 : Sum  Inputs=++++
  Bus Creator : BusCreator  Inputs=6
  Constant : Constant  Value=uavParam.geom.RotorArm1
  Constant1 : Constant  Value=0
  Constant10 : Constant  Value=uavParam.geom.RotorArm4
  Constant11 : Constant  Value=[0 0 -1]
  Constant13 : Constant  Value=[ 0; 0; 1]
  Constant2 : Constant  Value=0
  Constant3 : Constant  Value=uavParam.geom.RotorArm2
  Constant5 : Constant  Value=[ 0; 0; 1]
  Constant6 : Constant  Value=uavParam.geom.RotorArm3
  Constant7 : Constant  Value=[0 0 -1]
  Constant8 : Constant  Value=[ 0; 0; -1]
  Constant9 : Constant  Value=[ 0; 0; -1]
  Cos1 : Trigonometry  Operator=cos
  Cos2 : Trigonometry  Operator=cos
  Gain : Gain  Gain=-1
  Gain1 : Gain  Gain=-1
  Gain{2..7} (6 alike) : Gain  Gain=0
  Model{,1..3} (4 alike) : ModelReference  ModelNameDialog=PropellerDynamics.slx  ModelReferenceVersion=3.9
  Mux : Mux  Inputs=3
  Mux1 : Mux  Inputs=3
  Sin1 : Trigonometry
  Sin2 : Trigonometry
  Tilt Servo Dynamics : Subsystem
  Transfer Fcn{,1..3} (4 alike) : TransferFcn  Denominator=[0.1 1]
  RotorParameters : Outport
  M : Outport  Port=2
  F : Outport  Port=3
  wires:
  Transfer Fcn3/1 -> Gain7/1
  Transfer Fcn2/1 -> Gain4/1
  Transfer Fcn1/1 -> [w2]
  Transfer Fcn/1 -> [w1]
  Bus Element In2/1 -> Tilt Servo Dynamics/2(TiltB)
  Bus Element In1/1 -> Tilt Servo Dynamics/1(TiltA)
  Tilt Servo Dynamics/2(Tilt2) -> [RotorB], Cos2/1, Sin1/1
  Tilt Servo Dynamics/1(Tilt1) -> [RotorA], Sin2/1, Cos1/1
  Bus Element In5/1 -> Model3/1
  Bus Element In4/1 -> Model2/1
  Bus Element In3/1 -> Model1/1
  Bus Element In/1 -> Model/1
  [RotorB] -> Bus Creator/6  "Rotor B"
  [RotorA] -> Bus Creator/5  "Rotor A"
  Bus Creator/1 -> RotorParameters/1
  [w4] -> Bus Creator/4  "w4"
  [w3] -> Bus Creator/3  "w3"
  [w2] -> Bus Creator/2  "w2"
  [w1] -> Bus Creator/1  "w1"
  Model3/3 -> Transfer Fcn3/1
  Model2/3 -> Transfer Fcn2/1
  Model1/3 -> Transfer Fcn1/1
  Model/3 -> Transfer Fcn/1
  [M1] -> Add1/1
  [M2] -> Add1/2
  [M3] -> Add1/3
  Add1/1 -> M/1
  [M4] -> Add1/4
  [F4] -> Add/4
  [F3] -> Add/3
  [F2] -> Add/2
  [F1] -> Add/1
  Model3/2 -> Gain6/1
  In Bus Element7/1 -> Model3/3
  Constant11/1 -> Model3/5
  Constant13/1 -> Model3/6
  Constant10/1 -> Model3/4
  In Bus Element6/1 -> Model3/2
  Model3/1 -> Gain5/1
  Model2/2 -> Gain3/1
  In Bus Element5/1 -> Model2/3
  Constant7/1 -> Model2/5
  Constant9/1 -> Model2/6
  Constant6/1 -> Model2/4
  In Bus Element4/1 -> Model2/2
  Model2/1 -> Gain2/1
  Model1/2 -> [M2]
  In Bus Element3/1 -> Model1/3
  [TiltArm2] -> Model1/5
  Constant5/1 -> Model1/6
  Constant3/1 -> Model1/4
  In Bus Element2/1 -> Model1/2
  Model1/1 -> [F2]
  Model/2 -> [M1]
  Model/1 -> [F1]
  Constant8/1 -> Model/6
  Gain1/1 -> Mux1/3
  Add/1 -> F/1
  [TiltArm1] -> Model/5
  Mux1/1 -> [TiltArm2]
  Constant2/1 -> Mux1/2
  Sin1/1 -> Mux1/1
  Cos2/1 -> Gain1/1
  Mux/1 -> [TiltArm1]
  Gain/1 -> Mux/3
  Constant1/1 -> Mux/2
  Cos1/1 -> Gain/1
  Sin2/1 -> Mux/1
  Constant/1 -> Model/4
  In Bus Element1/1 -> Model/3
  In Bus Element/1 -> Model/2
  Gain2/1 -> [F3]
  Gain3/1 -> [M3]
  Gain4/1 -> [w3]
  Gain5/1 -> [F4]
  Gain6/1 -> [M4]
  Gain7/1 -> [w4]

== system Dynamics3/Digital Twin/Force and Moments/Weather Model ==
  AirData : Inport
  Xe : Inport  Port=2
  Euler : Inport  Port=3
  Simple Model : Subsystem  VariantControl=Wind==0
  Weather Model : Subsystem  VariantControl=Wind==1
  Wind_e : Outport
  Rho : Outport  Port=2

== system Dynamics3/Digital Twin/Force and Moments/Aerodynamic Forces/Compute Air Data ==
  Vb : Inport  PortDimensions=3
  Rho : Inport  Port=2
  Bus Creator : BusCreator  Inputs=4
  Dynamic Pressure : aerolibasang/Dynamic Pressure
  "Incidence, Sideslip, & Airspeed" : aerolibasang/Incidence, Sideslip, & Airspeed
  Saturation : Saturate  UpperLimit=14*pi/180  LowerLimit=-14*pi/180
  Scope : Scope
  AirData : Outport  VectorParamsAs1DForOutWhenUnconnected=off
  wires:
  Saturation/1 -> Bus Creator/2  "beta"
  "Incidence, Sideslip, & Airspeed"/2 -> Saturation/1  "beta"
  Vb/1 -> Dynamic Pressure/1, "Incidence, Sideslip, & Airspeed"/1
  Dynamic Pressure/1 -> Bus Creator/4  "q"
  "Incidence, Sideslip, & Airspeed"/3 -> Bus Creator/3  "airspeed"
  Rho/1 -> Dynamic Pressure/2
  "Incidence, Sideslip, & Airspeed"/1 -> Bus Creator/1  "alpha"
  Bus Creator/1 -> AirData/1, Scope/1

== system Dynamics3/Digital Twin/Force and Moments/Aerodynamic Forces/Compute Body Frame Forces and Moments ==
  AirData : Inport
  CtrlSurfaces : Inport  Port=2
  p,q,r : Inport  Port=3
  Bus Selector : BusSelector  OutputSignals=alpha,beta
  Mux : Mux  Inputs=2
  Rotate FM to body frame : Subsystem
  Wind frame F& M : Subsystem
  F_b : Outport  Unit=kg*m/s^2  VectorParamsAs1DForOutWhenUnconnected=off
  M_b : Outport  Port=2  Unit=kg*m/s  VectorParamsAs1DForOutWhenUnconnected=off
  wires:
  AirData/1 -> Bus Selector/1, Wind frame F& M/1(Airdata)
  CtrlSurfaces/1 -> Wind frame F& M/2(CtrlSurfaces)
  Rotate FM to body frame/1(F_b) -> F_b/1
  Rotate FM to body frame/2(M_b) -> M_b/1
  p,q,r/1 -> Wind frame F& M/3(p,q,r)
  Wind frame F& M/1(FM_w) -> Rotate FM to body frame/1(FM_w)  "FM_W"
  Bus Selector/1 -> Mux/1  "<alpha>"
  Bus Selector/2 -> Mux/2  "<beta>"
  Mux/1 -> Rotate FM to body frame/2(alpha_beta)

== system Dynamics3/Digital Twin/Force and Moments/Aerodynamic Forces/Rotate Vw ==
  Vw : Inport
  Euler : Inport  Port=2
  RL2B : mbdriLib/Coordinates/RL2B  SystemSampleTime=-1  VariantActivationTime=update diagram  AllowFlexibleInterface=on  Latency=0  AutoFrameSizeCalculation=off
  RL2B * Vw : Product  Multiplication=Matrix(*)  InputSameDT=on  SaturateOnIntegerOverflow=on  OutDataTypeStr=Inherit: Same as first input
  Vb : Outport  Unit=m/s  VectorParamsAs1DForOutWhenUnconnected=off
  wires:
  Euler/1 -> RL2B/1
  RL2B/1 -> RL2B * Vw/1
  Vw/1 -> RL2B * Vw/2
  RL2B * Vw/1 -> Vb/1

== system Dynamics3/Digital Twin/Force and Moments/Propulsion/Tilt Servo Dynamics ==
  TiltA : Inport
  TiltB : Inport  Port=2
  Gain2 : Gain  Gain=pi/2
  Gain3 : Gain  Gain=pi/2
  IC : InitialCondition  Value=tiltIni
  IC1 : InitialCondition  Value=tiltIni
  Servo Dynamics : TransferFcn  Denominator=[0.1 1]
  Servo Dynamics1 : TransferFcn  Denominator=[0.1 1]
  Tilt1 : Outport
  Tilt2 : Outport  Port=2
  wires:
  TiltA/1 -> Gain2/1
  Gain3/1 -> Servo Dynamics1/1
  IC1/1 -> Tilt1/1  "Tilt1"
  IC/1 -> Tilt2/1  "Tilt2"
  Servo Dynamics1/1 -> IC/1
  Servo Dynamics/1 -> IC1/1
  TiltB/1 -> Gain3/1
  Gain2/1 -> Servo Dynamics/1

== system Dynamics3/Digital Twin/Force and Moments/Weather Model/Simple Model ==
  AirData : Inport
  Xe : Inport  Port=2
  Euler : Inport  Port=3
  Constant : Constant  Value=[ 0 0 0]
      settings: AttributesFormatString=%<Value>
  Constant1 : Constant  Value=uavParam.aero.rho
  Terminator : Terminator
  Terminator1 : Terminator
  Terminator3 : Terminator
  Wind_e : Outport  Unit=m/s  VectorParamsAs1DForOutWhenUnconnected=off
  " Rho" : Outport  Port=2  VectorParamsAs1DForOutWhenUnconnected=off
  wires:
  Constant1/1 -> " Rho"/1
  Xe/1 -> Terminator3/1
  Euler/1 -> Terminator1/1
  Constant/1 -> Wind_e/1
  AirData/1 -> Terminator/1

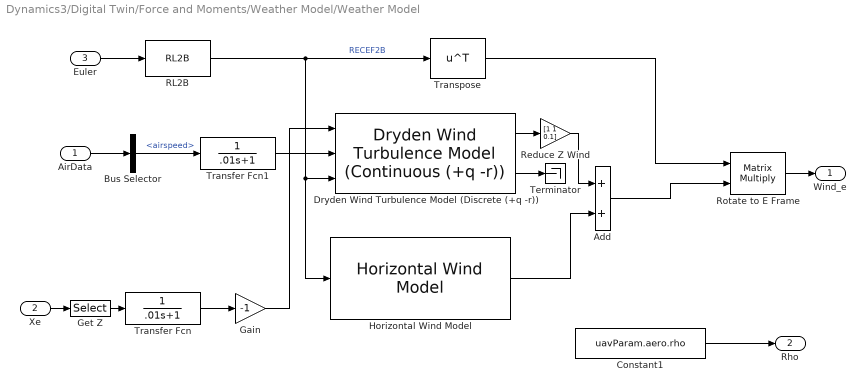
== system Dynamics3/Digital Twin/Force and Moments/Weather Model/Weather Model ==
  AirData : Inport
  Xe : Inport  Port=2
  Euler : Inport  Port=3
  Add : Sum  Inputs=2
  Bus Selector : BusSelector  OutputSignals=airspeed
  Constant1 : Constant  Value=uavParam.aero.rho
  Dryden Wind Turbulence Model (Discrete (+q -r)) : aerolibwind2/Dryden Wind Turbulence Model  (Continuous (+q -r))  units=Metric (MKS)  spec=MIL-F-8785C  model=Discrete Dryden (+q -r)  W20=env.windBase/4  Wdeg=env.windDirTurb  TurbProb=10^-2 - Light  L_high=533.4  Wingspan=uavParam.geom.b  ts=0.005  Seed=[23341 23342 23343 23344]  T_on=on
  Gain : Gain  Gain=-1
      settings: AttributesFormatString=Z to Alt
  Get Z : Selector  InputPortWidth=3  IndexOptions=Index vector (dialog)  Indices=[3]  OutputSizes=[(-2)]
  Horizontal Wind Model : aerolibwind2/Horizontal Wind Model  units=Metric (MKS)  Vw_source=Internal  Vwind=env.windBase  W_source=Internal  Wdeg=env.windDirHor
  RL2B : mbdriLib/Coordinates/RL2B  SystemSampleTime=-1  VariantActivationTime=update diagram  AllowFlexibleInterface=on  Latency=0  AutoFrameSizeCalculation=off
  Reduce Z Wind : Gain  Gain=[1 1 0.1]
      settings: AttributesFormatString=%<Gain>
  Rotate to E Frame : Product  Multiplication=Matrix(*)
  Terminator : Terminator
  Transfer Fcn : TransferFcn  Denominator=[.01 1]
  Transfer Fcn1 : TransferFcn  Denominator=[.01 1]
  Transpose : Math  Operator=transpose  SignedPower=on
  Wind_e : Outport  Unit=m/s  VectorParamsAs1DForOutWhenUnconnected=off
  Rho : Outport  Port=2  VectorParamsAs1DForOutWhenUnconnected=off
  wires:
  Constant1/1 -> Rho/1
  Gain/1 -> Dryden Wind Turbulence Model (Discrete (+q -r))/1
  Xe/1 -> Get Z/1
  Get Z/1 -> Transfer Fcn/1
  Euler/1 -> RL2B/1
  RL2B/1 -> Transpose/1, Horizontal Wind Model/1, Dryden Wind Turbulence Model (Discrete (+q -r))/3  "RECEF2B"
  Add/1 -> Rotate to E Frame/2
  Transfer Fcn1/1 -> Dryden Wind Turbulence Model (Discrete (+q -r))/2
  Horizontal Wind Model/1 -> Add/2
  Transpose/1 -> Rotate to E Frame/1
  Rotate to E Frame/1 -> Wind_e/1
  Dryden Wind Turbulence Model (Discrete (+q -r))/1 -> Reduce Z Wind/1
  Reduce Z Wind/1 -> Add/1
  Dryden Wind Turbulence Model (Discrete (+q -r))/2 -> Terminator/1
  Transfer Fcn/1 -> Gain/1
  AirData/1 -> Bus Selector/1
  Bus Selector/1 -> Transfer Fcn1/1  "<airspeed>"

== system Dynamics3/Digital Twin/Force and Moments/Aerodynamic Forces/Compute Body Frame Forces and Moments/Rotate FM to body frame ==
  FM_w : Inport
  alpha_beta : Inport  Port=2
  Forces : Selector  InputPortWidth=6  IndexOptions=Index vector (dialog)  Indices=[1 2 3]  OutputSizes=[(-2)]
  Moments : Selector  InputPortWidth=6  IndexOptions=Index vector (dialog)  Indices=[4 5 6]  OutputSizes=[(-2)]
  Rotate Forces : Subsystem
  Rotate Moments : Subsystem
  F_b : Outport  VectorParamsAs1DForOutWhenUnconnected=off
  M_b : Outport  Port=2  VectorParamsAs1DForOutWhenUnconnected=off
  wires:
  Rotate Forces/1(F_b) -> F_b/1
  Rotate Moments/1(M_b) -> M_b/1
  Forces/1 -> Rotate Forces/1(F_w)
  FM_w/1 -> Forces/1, Moments/1
  Moments/1 -> Rotate Moments/2(M_w)
  alpha_beta/1 -> Rotate Moments/1(alpha_beta), Rotate Forces/2(alpha_beta)

== system Dynamics3/Digital Twin/Force and Moments/Aerodynamic Forces/Compute Body Frame Forces and Moments/Wind frame F& M ==
  Airdata : Inport
  CtrlSurfaces : Inport  Port=2
  p,q,r : Inport  Port=3
  Bus Creator1 : BusCreator  Inputs=2
  Bus Selector1 : BusSelector  OutputSignals=dA,dR
  Bus Selector2 : BusSelector  OutputSignals=dE,dA,dR
  Bus Selector6 : BusSelector  OutputSignals=beta,airspeed
  Bus Selector7 : BusSelector  OutputSignals=alpha,airspeed
  Get Forces and Moments : Subsystem
  Lateral Channel : Subsystem
  Longitudinal Channel : Subsystem
  FM_w : Outport  PortDimensions=6  VectorParamsAs1DForOutWhenUnconnected=off
  wires:
  Bus Selector2/3 -> Longitudinal Channel/6(dR)  "<dR>"
  Bus Selector2/2 -> Longitudinal Channel/5(dA)  "<dA>"
  Longitudinal Channel/1(Longitudinal) -> Bus Creator1/2
  Lateral Channel/1(Lateral) -> Bus Creator1/1
  p,q,r/1 -> Longitudinal Channel/4(p,q,r), Lateral Channel/5(p,q,r)
  CtrlSurfaces/1 -> Bus Selector2/1, Bus Selector1/1
  Bus Selector1/1 -> Lateral Channel/3(dA)  "<dA>"
  Bus Selector1/2 -> Lateral Channel/4(dR)  "<dR>"
  Bus Selector2/1 -> Longitudinal Channel/3(dE)  "<dE>"
  Airdata/1 -> Get Forces and Moments/1(Airdata), Bus Selector7/1, Bus Selector6/1
  Bus Selector6/1 -> Lateral Channel/1(beta)  "<beta>"
  Bus Selector6/2 -> Lateral Channel/2(Airspeed)  "<airspeed>"
  Bus Selector7/1 -> Longitudinal Channel/1(alpha)  "<alpha>"
  Bus Selector7/2 -> Longitudinal Channel/2(Airpseed)  "<airspeed>"
  Bus Creator1/1 -> Get Forces and Moments/2(AeroCoeffs)
  Get Forces and Moments/1(FM_w) -> FM_w/1

== system Dynamics3/Digital Twin/Force and Moments/Aerodynamic Forces/Compute Body Frame Forces and Moments/Rotate FM to body frame/Rotate Forces ==
  F_w : Inport
  alpha_beta : Inport  Port=2
  Product2 : Product  Multiplication=Matrix(*)  SaturateOnIntegerOverflow=on  OutDataTypeStr=Inherit: Same as first input
  RB2W : Subsystem
  RW2B : Math  Operator=transpose  SignedPower=on
  F_b : Outport  PortDimensions=3  VectorParamsAs1DForOutWhenUnconnected=off
  wires:
  RB2W/1(Rw2b) -> RW2B/1
  alpha_beta/1 -> RB2W/1(aoa beta)
  Product2/1 -> F_b/1
  F_w/1 -> Product2/2
  RW2B/1 -> Product2/1

== system Dynamics3/Digital Twin/Force and Moments/Aerodynamic Forces/Compute Body Frame Forces and Moments/Rotate FM to body frame/Rotate Moments ==
  alpha_beta : Inport
  M_w : Inport  Port=2
  Product2 : Product  Multiplication=Matrix(*)  SaturateOnIntegerOverflow=on  OutDataTypeStr=Inherit: Same as first input
  RB2W : Subsystem
  RW2B : Math  Operator=transpose  SignedPower=on
  M_b : Outport  PortDimensions=3  VectorParamsAs1DForOutWhenUnconnected=off
  wires:
  M_w/1 -> Product2/2
  Product2/1 -> M_b/1
  alpha_beta/1 -> RB2W/1(aoa beta)
  RB2W/1(Rw2b) -> RW2B/1
  RW2B/1 -> Product2/1

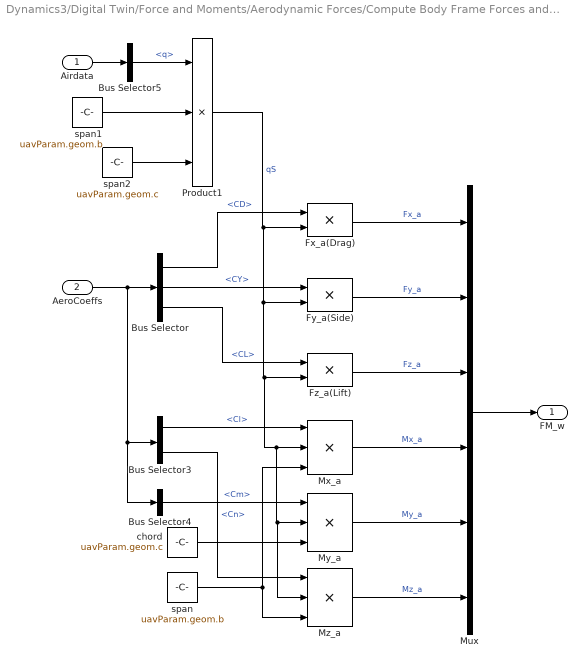
== system Dynamics3/Digital Twin/Force and Moments/Aerodynamic Forces/Compute Body Frame Forces and Moments/Wind frame F& M/Get Forces and Moments ==
  Airdata : Inport
  AeroCoeffs : Inport  Port=2
  Bus Selector : BusSelector  OutputSignals=signal2.CD,signal1.CY,signal2.CL
  Bus Selector3 : BusSelector  OutputSignals=signal1.Cl,signal1.Cn
  Bus Selector4 : BusSelector  OutputSignals=signal2.Cm
  Bus Selector5 : BusSelector  OutputSignals=q
  Fx_a(Drag) : Product  Inputs=**  SaturateOnIntegerOverflow=on  OutDataTypeStr=Inherit: Same as first input
  Fy_a(Side) : Product  SaturateOnIntegerOverflow=on  OutDataTypeStr=Inherit: Same as first input
  Fz_a(Lift) : Product  SaturateOnIntegerOverflow=on  OutDataTypeStr=Inherit: Same as first input
  Mux : Mux  Inputs=6
  Mx_a : Product  Inputs=3  SaturateOnIntegerOverflow=on  OutDataTypeStr=Inherit: Same as first input
  My_a : Product  Inputs=3  SaturateOnIntegerOverflow=on  OutDataTypeStr=Inherit: Same as first input
  Mz_a : Product  Inputs=3  SaturateOnIntegerOverflow=on  OutDataTypeStr=Inherit: Same as first input
  Product1 : Product  Inputs=3  SaturateOnIntegerOverflow=on  OutDataTypeStr=Inherit: Same as first input
  chord : Constant  Value=uavParam.geom.c  VectorParams1D=off
      settings: AttributesFormatString=%<Value>
  span : Constant  Value=uavParam.geom.b  VectorParams1D=off
      settings: AttributesFormatString=%<Value>
  span1 : Constant  Value=uavParam.geom.b  VectorParams1D=off
      settings: AttributesFormatString=%<Value>
  span2 : Constant  Value=uavParam.geom.c  VectorParams1D=off
      settings: AttributesFormatString=%<Value>
  FM_w : Outport  VectorParamsAs1DForOutWhenUnconnected=off
  wires:
  Bus Selector5/1 -> Product1/1  "<q>"
  Bus Selector3/1 -> Mx_a/1  "<Cl>"
  span1/1 -> Product1/2
  Product1/1 -> Mz_a/2, My_a/2, Mx_a/2, Fz_a(Lift)/2, Fy_a(Side)/2, Fx_a(Drag)/2  "qS"
  Bus Selector/3 -> Fz_a(Lift)/1  "<CL>"
  Bus Selector3/2 -> Mz_a/1  "<Cn>"
  Mux/1 -> FM_w/1
  Fy_a(Side)/1 -> Mux/2  "Fy_a"
  span/1 -> Mx_a/3, Mz_a/3
  chord/1 -> My_a/3
  Airdata/1 -> Bus Selector5/1
  Mz_a/1 -> Mux/6  "Mz_a"
  Fz_a(Lift)/1 -> Mux/3  "Fz_a"
  My_a/1 -> Mux/5  "My_a"
  AeroCoeffs/1 -> Bus Selector3/1, Bus Selector4/1, Bus Selector/1
  Bus Selector/1 -> Fx_a(Drag)/1  "<CD>"
  Fx_a(Drag)/1 -> Mux/1  "Fx_a"
  span2/1 -> Product1/3
  Bus Selector4/1 -> My_a/1  "<Cm>"
  Bus Selector/2 -> Fy_a(Side)/1  "<CY>"
  Mx_a/1 -> Mux/4  "Mx_a"

== system Dynamics3/Digital Twin/Force and Moments/Aerodynamic Forces/Compute Body Frame Forces and Moments/Wind frame F& M/Lateral Channel ==
  beta : Inport
  Airspeed : Inport  Port=2
  dA : Inport  Port=3
  dR : Inport  Port=4
  p,q,r : Inport  Port=5
  Bus Creator : BusCreator  Inputs=3
  CY : Subsystem
  Cl : Subsystem
  Cn : Subsystem
  Lateral : Outport  VectorParamsAs1DForOutWhenUnconnected=off
  wires:
  Bus Creator/1 -> Lateral/1
  CY/1(CY) -> Bus Creator/1  "CY"
  Cn/1(Cn) -> Bus Creator/3  "Cn"
  beta/1 -> Cn/1(beta), Cl/1(beta), CY/1(beta)
  dA/1 -> Cn/2(dA), Cl/2(dA)
  dR/1 -> Cn/3(dR), Cl/3(dR), CY/2(dR)
  Airspeed/1 -> Cl/5(Airspeed), Cn/5(Airspeed), CY/4(Airspeed)
  p,q,r/1 -> Cl/4(p,q,r), Cn/4(p,q,r), CY/3(p,q,r)
  Cl/1(Cl) -> Bus Creator/2  "Cl"

== system Dynamics3/Digital Twin/Force and Moments/Aerodynamic Forces/Compute Body Frame Forces and Moments/Wind frame F& M/Longitudinal Channel ==
  alpha : Inport
  Airpseed : Inport  Port=2
  dE : Inport  Port=3
  p,q,r : Inport  Port=4
  dA : Inport  Port=5
  dR : Inport  Port=6
  Bus Creator : BusCreator  Inputs=3
  CD : Subsystem
  CL : Subsystem
  Cm : Subsystem
  Saturation : Saturate  UpperLimit=14*pi/180  LowerLimit=-14*pi/180
  Y-down : Gain  Gain=-1  SaturateOnIntegerOverflow=on  OutDataTypeStr=Inherit: Same as input  ParamDataTypeStr=Inherit: Same as input
      settings: AttributesFormatString=%<Gain>
  alpha_dot : TransferFcn  Numerator=[1 0]  Denominator=[0.1 1]
  Longitudinal : Outport  VectorParamsAs1DForOutWhenUnconnected=off
  wires:
  Saturation/1 -> CL/1(alpha), Cm/1(alpha), alpha_dot/1
  dA/1 -> CL/6(dA), CD/2(dA)
  dR/1 -> CD/3(dR)
  alpha/1 -> Saturation/1
  CD/1(CD) -> Bus Creator/1  "CD"
  Y-down/1 -> Bus Creator/2  "CL"
  dE/1 -> CL/3(dE), CD/4(dE), Cm/2(De)
  CL/1(CL) -> Y-down/1, CD/1(CL)
  Cm/1(Cm) -> Bus Creator/3  "Cm"
  Bus Creator/1 -> Longitudinal/1
  p,q,r/1 -> CL/4(p,q,r), Cm/3(p,q,r)
  Airpseed/1 -> CL/5(Airspeed), Cm/4(Airspeed)
  alpha_dot/1 -> CL/2(alpha_dot)
